simulink model "model2"  (R2020b)
settings: Solver=VariableStepAuto  StartTime=0.0  StopTime=10.0  RelTol=1e-3
settings Model: Creator=dkravchenko  LastModifiedBy=dkravchenko

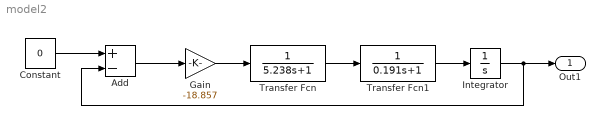
== system model2 ==
  Add : Sum  Inputs=+-
  Constant : Constant  Value=0
  Gain : Gain  Gain=-18.857
  Integrator : Integrator
  Transfer Fcn : TransferFcn  Denominator=[5.238 1]
  Transfer Fcn1 : TransferFcn  Denominator=[0.191 1]
  Out1 : Outport
  wires:
  Constant/1 -> Add/1
  Add/1 -> Gain/1
  Gain/1 -> Transfer Fcn/1
  Transfer Fcn/1 -> Transfer Fcn1/1
  Transfer Fcn1/1 -> Integrator/1
  Integrator/1 -> Add/2, Out1/1
